simulink model "echantillonnage_simple"  (Simulink 6.2)
settings: Solver=FixedStepDiscrete  StartTime=0.0  StopTime=t_sim  FixedStep=ts  RelTol=1e-3
values from neighbouring files (symbols this model uses):
  ts = 0.000001    (= 1e-06)    [main.m]
settings Model: LastModifiedBy=Mailly
settings DebuggingCC: SolverPrmCheckMsg=warning

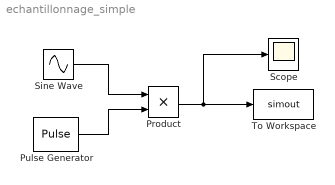
== system echantillonnage_simple ==
  Product : Product  SampleTime=0  RndMeth=Zero
  Pulse Generator : DiscretePulseGenerator  Period=1000  PulseWidth=200  SampleTime=ts
  Scope : Scope
      settings: YMin=-1.5  YMax=1.5
  Sine Wave : Sin  Frequency=2*pi*100  SampleTime=ts
  To Workspace : ToWorkspace  VariableName=simout  SampleTime=ts  SaveFormat=Array
  wires:
  Sine Wave/1 -> Product/1
  Product/1 -> To Workspace/1, Scope/1
  Pulse Generator/1 -> Product/2
